simulink model "ThdRwLtStFwdBkwdTrgtPosSelc"  (R2018b)
settings: Solver=FixedStepDiscrete  StartTime=0.0  StopTime=10.0  FixedStep=0.01  RelTol=1e-3
undefined symbols (not defined in the file or in its folder): KeSMSw6sAcsEntryThdRwLtStFrwdBkwdPos_Val, KeSMSw6sAcsEntryThdRwLtStFrwdBkwdPosMax_Val, KeSMSw6sAcsEntryThdRwLtStFrwdBkwdPosMin_Val, KeSMSw6sFamilyLMdThdRwLtStFrwdBkwdPos_Val, KeSMSw6sFamilyLMdThdRwLtStFrwdBkwdPosMax_Val, KeSMSw6sFamilyLMdThdRwLtStFrwdBkwdPosMin_Val, KeSMSw6sFamilyMdThdRwLtStFrwdBkwdPos_Val, KeSMSw6sFamilyMdThdRwLtStFrwdBkwdPosMax_Val, KeSMSw6sFamilyMdThdRwLtStFrwdBkwdPosMin_Val, KeSMSw6sLugThdRwLtStFrwdBkwdPos_Val, KeSMSw6sLugThdRwLtStFrwdBkwdPosMax_Val, KeSMSw6sLugThdRwLtStFrwdBkwdPosMin_Val, KeSMSw6sVIPThdRwLtStFrwdBkwdPos_Val, KeSMSw6sVIPThdRwLtStFrwdBkwdPosMax_Val, KeSMSw6sVIPThdRwLtStFrwdBkwdPosMin_Val, KeSMSwAcsEntryThdRwLtStFrwdBkwdPos_Val, KeSMSwAcsEntryThdRwLtStFrwdBkwdPosMax_Val, KeSMSwAcsEntryThdRwLtStFrwdBkwdPosMin_Val, KeSMSwFamilyLMdThdRwLtStFrwdBkwdPos_Val, KeSMSwFamilyLMdThdRwLtStFrwdBkwdPosMax_Val, KeSMSwFamilyLMdThdRwLtStFrwdBkwdPosMin_Val, KeSMSwFamilyMdThdRwLtStFrwdBkwdPos_Val, KeSMSwFamilyMdThdRwLtStFrwdBkwdPosMax_Val, KeSMSwFamilyMdThdRwLtStFrwdBkwdPosMin_Val, KeSMSwLugThdRwLtStFrwdBkwdPos_Val, KeSMSwLugThdRwLtStFrwdBkwdPosMax_Val, KeSMSwLugThdRwLtStFrwdBkwdPosMin_Val, KeSMSwVIPThdRwLtStFrwdBkwdPos_Val, KeSMSwVIPThdRwLtStFrwdBkwdPosMax_Val, KeSMSwVIPThdRwLtStFrwdBkwdPosMin_Val
libraries: TrgtPosSelcLib x6
settings Model: Creator=sn2xws  LastModifiedBy=sn2xws
settings Model: ModifiedHistory=|
  | V2.1.0 Bug 540874 将外部标定改为固定值0
  | 2024.7.5 V3.0.0 557模式流程V1.9
settings DataIOCC: SaveFormat=StructureWithTime
settings OptimizationCC: DefaultParameterBehavior=Inlined  EnhancedBackFolding=on  PassReuseOutputArgsAs=Individual arguments  ZeroExternalMemoryAtStartup=off  ZeroInternalMemoryAtStartup=off  OptimizeBlockOrder=speed  DifferentSizesBufferReuse=on  OptimizationCustomize=off
settings DebuggingCC: ParameterTunabilityLossMsg=error
settings SFSimCC: MATLABDynamicMemAlloc=off
settings RTWCC: SystemTargetFile=autosar.tlc  GenCodeOnly=on  TemplateMakefile=ert_default_tmf  Description=AUTOSAR  GenerateReport=on  IncludeHyperlinkInReport=on  LaunchReport=on  GenerateTraceInfo=on  GenerateTraceReport=on  GenerateTraceReportSl=on  GenerateTraceReportSf=on  GenerateTraceReportEml=on  GenerateCodeMetricsReport=on
settings CodeAppCC: ForceParamTrailComments=on  IgnoreCustomStorageClasses=off  OperatorAnnotations=on  SimulinkDataObjDesc=on  SFDataObjDesc=on  InsertBlockDesc=on
settings STFCustomTargetCC: TargetLangStandard=C99 (ISO)  MultiwordLength=256  ParMdlRefBuildCompliant=on  CompOptLevelCompliant=on  IncludeMdlTerminateFcn=off  CombineOutputUpdateFcns=on  SuppressErrorStatus=on  ERTCustomFileBanners=on  SupportNonFinite=off  SupportComplex=off  SupportContinuousTime=off  SupportNonInlinedSFcns=off  RemoveResetFunc=on  MATLABClassNameForMDSCustomization=Simulink.SoftwareTarget.ERTCustomization  AutosarCompliant=on  UseToolchainInfoCompliant=on  LookupTableObjectStructAxisOrder=2,1,3,4,...  LUTObjectStructOrderEvenSpacing=Size,Table,Breakpoints  SystemTargetFile=autosar.tlc
settings ERTTargetCC: TargetLangStandard=C99 (ISO)  ConcurrentExecutionCompliant=off  IncludeMdlTerminateFcn=off  SuppressErrorStatus=on  SupportNonFinite=off  SupportComplex=off  ModelStepFunctionPrototypeControlCompliant=off  CPPClassGenCompliant=off  AutosarCompliant=on  LookupTableObjectStructAxisOrder=2,1,3,4,...  LUTObjectStructOrderEvenSpacing=Size,Table,Breakpoints  InlinedParameterPlacement=NonHierarchical  ERTCustomFileTemplate=example_file_process.tlc  ERTFilePackagingFormat=Compact

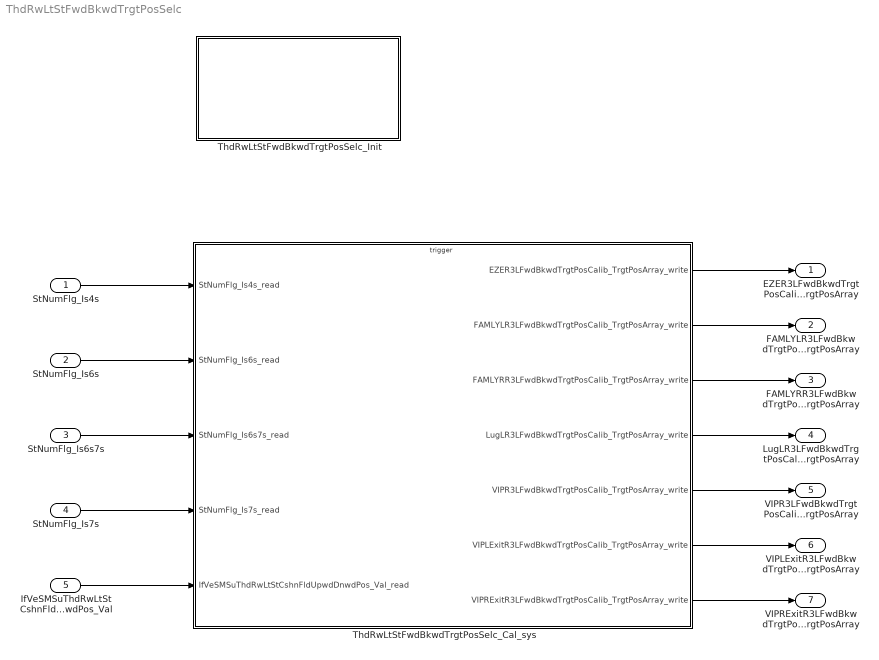
== system ThdRwLtStFwdBkwdTrgtPosSelc ==
  StNumFlg_Is4s : Inport  OutDataTypeStr=boolean  PortDimensions=1
  StNumFlg_Is6s : Inport  Port=2  OutDataTypeStr=boolean  PortDimensions=1
  StNumFlg_Is6s7s : Inport  Port=3  OutDataTypeStr=boolean  PortDimensions=1
  StNumFlg_Is7s : Inport  Port=4  OutDataTypeStr=boolean  PortDimensions=1
  IfVeSMSuThdRwLtStCshnFldUpwdDnwdPos_Val : Inport  Port=5  OutDataTypeStr=uint16  PortDimensions=1
  ThdRwLtStFwdBkwdTrgtPosSelc_Cal_sys : Subsystem
  ThdRwLtStFwdBkwdTrgtPosSelc_Init : Subsystem
  EZER3LFwdBkwdTrgtPosCalib_TrgtPosArray : Outport  Description=|  OutDataTypeStr=uint16  PortDimensions=3
      | 0:Pos
      | 1:Max
      | 2:Min
  FAMLYLR3LFwdBkwdTrgtPosCalib_TrgtPosArray : Outport  Description=|  Port=2  OutDataTypeStr=uint16  PortDimensions=3
      | 0:Pos
      | 1:Max
      | 2:Min
  FAMLYRR3LFwdBkwdTrgtPosCalib_TrgtPosArray : Outport  Description=|  Port=3  OutDataTypeStr=uint16  PortDimensions=3
      | 0:Pos
      | 1:Max
      | 2:Min
  LugLR3LFwdBkwdTrgtPosCalib_TrgtPosArray : Outport  Description=|  Port=4  OutDataTypeStr=uint16  PortDimensions=3
      | 0:Pos
      | 1:Max
      | 2:Min
  VIPR3LFwdBkwdTrgtPosCalib_TrgtPosArray : Outport  Description=|  Port=5  OutDataTypeStr=uint16  PortDimensions=3
      | 0:Pos
      | 1:Max
      | 2:Min
  VIPLExitR3LFwdBkwdTrgtPosCalib_TrgtPosArray : Outport  Description=|  Port=6  OutDataTypeStr=uint16  PortDimensions=3
      | 0:Pos
      | 1:Max
      | 2:Min
  VIPRExitR3LFwdBkwdTrgtPosCalib_TrgtPosArray : Outport  Description=|  Port=7  OutDataTypeStr=uint16  PortDimensions=3
      | 0:Pos
      | 1:Max
      | 2:Min
  wires:
  StNumFlg_Is4s/1 -> ThdRwLtStFwdBkwdTrgtPosSelc_Cal_sys/1(StNumFlg_Is4s_read)
  StNumFlg_Is6s/1 -> ThdRwLtStFwdBkwdTrgtPosSelc_Cal_sys/2(StNumFlg_Is6s_read)
  StNumFlg_Is6s7s/1 -> ThdRwLtStFwdBkwdTrgtPosSelc_Cal_sys/3(StNumFlg_Is6s7s_read)
  StNumFlg_Is7s/1 -> ThdRwLtStFwdBkwdTrgtPosSelc_Cal_sys/4(StNumFlg_Is7s_read)
  ThdRwLtStFwdBkwdTrgtPosSelc_Cal_sys/1(EZER3LFwdBkwdTrgtPosCalib_TrgtPosArray_write) -> EZER3LFwdBkwdTrgtPosCalib_TrgtPosArray/1
  ThdRwLtStFwdBkwdTrgtPosSelc_Cal_sys/2(FAMLYLR3LFwdBkwdTrgtPosCalib_TrgtPosArray_write) -> FAMLYLR3LFwdBkwdTrgtPosCalib_TrgtPosArray/1
  ThdRwLtStFwdBkwdTrgtPosSelc_Cal_sys/3(FAMLYRR3LFwdBkwdTrgtPosCalib_TrgtPosArray_write) -> FAMLYRR3LFwdBkwdTrgtPosCalib_TrgtPosArray/1
  ThdRwLtStFwdBkwdTrgtPosSelc_Cal_sys/4(LugLR3LFwdBkwdTrgtPosCalib_TrgtPosArray_write) -> LugLR3LFwdBkwdTrgtPosCalib_TrgtPosArray/1
  ThdRwLtStFwdBkwdTrgtPosSelc_Cal_sys/5(VIPR3LFwdBkwdTrgtPosCalib_TrgtPosArray_write) -> VIPR3LFwdBkwdTrgtPosCalib_TrgtPosArray/1
  ThdRwLtStFwdBkwdTrgtPosSelc_Cal_sys/6(VIPLExitR3LFwdBkwdTrgtPosCalib_TrgtPosArray_write) -> VIPLExitR3LFwdBkwdTrgtPosCalib_TrgtPosArray/1
  ThdRwLtStFwdBkwdTrgtPosSelc_Cal_sys/7(VIPRExitR3LFwdBkwdTrgtPosCalib_TrgtPosArray_write) -> VIPRExitR3LFwdBkwdTrgtPosCalib_TrgtPosArray/1
  IfVeSMSuThdRwLtStCshnFldUpwdDnwdPos_Val/1 -> ThdRwLtStFwdBkwdTrgtPosSelc_Cal_sys/5(IfVeSMSuThdRwLtStCshnFldUpwdDnwdPos_Val_read)

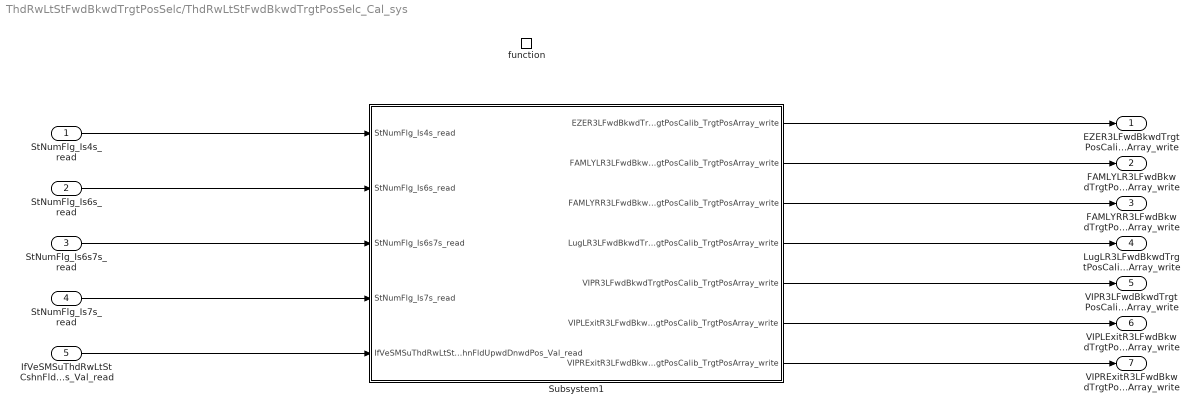
== system ThdRwLtStFwdBkwdTrgtPosSelc/ThdRwLtStFwdBkwdTrgtPosSelc_Cal_sys ==
  StNumFlg_Is4s_read : Inport
  StNumFlg_Is6s_read : Inport  Port=2
  StNumFlg_Is6s7s_read : Inport  Port=3
  StNumFlg_Is7s_read : Inport  Port=4
  IfVeSMSuThdRwLtStCshnFldUpwdDnwdPos_Val_read : Inport  Port=5
  function : TriggerPort  TriggerType=function-call  IsSimulinkFunction=on  FunctionName=ThdRwLtStFwdBkwdTrgtPosSelc_Cal  VariantControl=(inherit)
  Subsystem1 : Subsystem
  EZER3LFwdBkwdTrgtPosCalib_TrgtPosArray_write : Outport
      settings: EnsureOutportIsVirtual=on
  FAMLYLR3LFwdBkwdTrgtPosCalib_TrgtPosArray_write : Outport  Port=2
      settings: EnsureOutportIsVirtual=on
  FAMLYRR3LFwdBkwdTrgtPosCalib_TrgtPosArray_write : Outport  Port=3
      settings: EnsureOutportIsVirtual=on
  LugLR3LFwdBkwdTrgtPosCalib_TrgtPosArray_write : Outport  Port=4
      settings: EnsureOutportIsVirtual=on
  VIPR3LFwdBkwdTrgtPosCalib_TrgtPosArray_write : Outport  Port=5
      settings: EnsureOutportIsVirtual=on
  VIPLExitR3LFwdBkwdTrgtPosCalib_TrgtPosArray_write : Outport  Port=6
      settings: EnsureOutportIsVirtual=on
  VIPRExitR3LFwdBkwdTrgtPosCalib_TrgtPosArray_write : Outport  Port=7
      settings: EnsureOutportIsVirtual=on
  wires:
  Subsystem1/1(EZER3LFwdBkwdTrgtPosCalib_TrgtPosArray_write) -> EZER3LFwdBkwdTrgtPosCalib_TrgtPosArray_write/1
  Subsystem1/2(FAMLYLR3LFwdBkwdTrgtPosCalib_TrgtPosArray_write) -> FAMLYLR3LFwdBkwdTrgtPosCalib_TrgtPosArray_write/1
  Subsystem1/3(FAMLYRR3LFwdBkwdTrgtPosCalib_TrgtPosArray_write) -> FAMLYRR3LFwdBkwdTrgtPosCalib_TrgtPosArray_write/1
  Subsystem1/4(LugLR3LFwdBkwdTrgtPosCalib_TrgtPosArray_write) -> LugLR3LFwdBkwdTrgtPosCalib_TrgtPosArray_write/1
  Subsystem1/5(VIPR3LFwdBkwdTrgtPosCalib_TrgtPosArray_write) -> VIPR3LFwdBkwdTrgtPosCalib_TrgtPosArray_write/1
  StNumFlg_Is4s_read/1 -> Subsystem1/1(StNumFlg_Is4s_read)
  StNumFlg_Is6s_read/1 -> Subsystem1/2(StNumFlg_Is6s_read)
  StNumFlg_Is6s7s_read/1 -> Subsystem1/3(StNumFlg_Is6s7s_read)
  StNumFlg_Is7s_read/1 -> Subsystem1/4(StNumFlg_Is7s_read)
  Subsystem1/6(VIPLExitR3LFwdBkwdTrgtPosCalib_TrgtPosArray_write) -> VIPLExitR3LFwdBkwdTrgtPosCalib_TrgtPosArray_write/1
  Subsystem1/7(VIPRExitR3LFwdBkwdTrgtPosCalib_TrgtPosArray_write) -> VIPRExitR3LFwdBkwdTrgtPosCalib_TrgtPosArray_write/1
  IfVeSMSuThdRwLtStCshnFldUpwdDnwdPos_Val_read/1 -> Subsystem1/5(IfVeSMSuThdRwLtStCshnFldUpwdDnwdPos_Val_read)

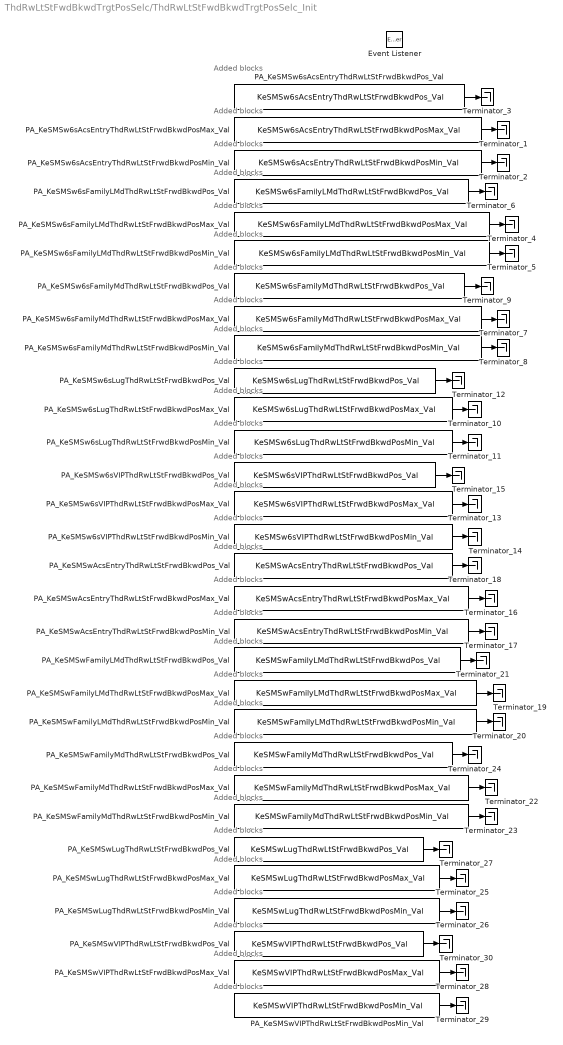
== system ThdRwLtStFwdBkwdTrgtPosSelc/ThdRwLtStFwdBkwdTrgtPosSelc_Init ==
  note: Added blocks
  note: Added blocks
  note: Added blocks
  note: Added blocks
  note: Added blocks
  note: Added blocks
  note: Added blocks
  note: Added blocks
  note: Added blocks
  note: Added blocks
  note: Added blocks
  note: Added blocks
  note: Added blocks
  note: Added blocks
  note: Added blocks
  note: Added blocks
  note: Added blocks
  note: Added blocks
  note: Added blocks
  note: Added blocks
  note: Added blocks
  note: Added blocks
  note: Added blocks
  note: Added blocks
  note: Added blocks
  note: Added blocks
  note: Added blocks
  note: Added blocks
  note: Added blocks
  note: Added blocks
  Event Listener : EventListener  EventName=reset
  PA_KeSMSw6sAcsEntryThdRwLtStFrwdBkwdPosMax_Val : Constant  Value=KeSMSw6sAcsEntryThdRwLtStFrwdBkwdPosMax_Val
  PA_KeSMSw6sAcsEntryThdRwLtStFrwdBkwdPosMin_Val : Constant  Value=KeSMSw6sAcsEntryThdRwLtStFrwdBkwdPosMin_Val
  PA_KeSMSw6sAcsEntryThdRwLtStFrwdBkwdPos_Val : Constant  Value=KeSMSw6sAcsEntryThdRwLtStFrwdBkwdPos_Val
  PA_KeSMSw6sFamilyLMdThdRwLtStFrwdBkwdPosMax_Val : Constant  Value=KeSMSw6sFamilyLMdThdRwLtStFrwdBkwdPosMax_Val
  PA_KeSMSw6sFamilyLMdThdRwLtStFrwdBkwdPosMin_Val : Constant  Value=KeSMSw6sFamilyLMdThdRwLtStFrwdBkwdPosMin_Val
  PA_KeSMSw6sFamilyLMdThdRwLtStFrwdBkwdPos_Val : Constant  Value=KeSMSw6sFamilyLMdThdRwLtStFrwdBkwdPos_Val
  PA_KeSMSw6sFamilyMdThdRwLtStFrwdBkwdPosMax_Val : Constant  Value=KeSMSw6sFamilyMdThdRwLtStFrwdBkwdPosMax_Val
  PA_KeSMSw6sFamilyMdThdRwLtStFrwdBkwdPosMin_Val : Constant  Value=KeSMSw6sFamilyMdThdRwLtStFrwdBkwdPosMin_Val
  PA_KeSMSw6sFamilyMdThdRwLtStFrwdBkwdPos_Val : Constant  Value=KeSMSw6sFamilyMdThdRwLtStFrwdBkwdPos_Val
  PA_KeSMSw6sLugThdRwLtStFrwdBkwdPosMax_Val : Constant  Value=KeSMSw6sLugThdRwLtStFrwdBkwdPosMax_Val
  PA_KeSMSw6sLugThdRwLtStFrwdBkwdPosMin_Val : Constant  Value=KeSMSw6sLugThdRwLtStFrwdBkwdPosMin_Val
  PA_KeSMSw6sLugThdRwLtStFrwdBkwdPos_Val : Constant  Value=KeSMSw6sLugThdRwLtStFrwdBkwdPos_Val
  PA_KeSMSw6sVIPThdRwLtStFrwdBkwdPosMax_Val : Constant  Value=KeSMSw6sVIPThdRwLtStFrwdBkwdPosMax_Val
  PA_KeSMSw6sVIPThdRwLtStFrwdBkwdPosMin_Val : Constant  Value=KeSMSw6sVIPThdRwLtStFrwdBkwdPosMin_Val
  PA_KeSMSw6sVIPThdRwLtStFrwdBkwdPos_Val : Constant  Value=KeSMSw6sVIPThdRwLtStFrwdBkwdPos_Val
  PA_KeSMSwAcsEntryThdRwLtStFrwdBkwdPosMax_Val : Constant  Value=KeSMSwAcsEntryThdRwLtStFrwdBkwdPosMax_Val
  PA_KeSMSwAcsEntryThdRwLtStFrwdBkwdPosMin_Val : Constant  Value=KeSMSwAcsEntryThdRwLtStFrwdBkwdPosMin_Val
  PA_KeSMSwAcsEntryThdRwLtStFrwdBkwdPos_Val : Constant  Value=KeSMSwAcsEntryThdRwLtStFrwdBkwdPos_Val
  PA_KeSMSwFamilyLMdThdRwLtStFrwdBkwdPosMax_Val : Constant  Value=KeSMSwFamilyLMdThdRwLtStFrwdBkwdPosMax_Val
  PA_KeSMSwFamilyLMdThdRwLtStFrwdBkwdPosMin_Val : Constant  Value=KeSMSwFamilyLMdThdRwLtStFrwdBkwdPosMin_Val
  PA_KeSMSwFamilyLMdThdRwLtStFrwdBkwdPos_Val : Constant  Value=KeSMSwFamilyLMdThdRwLtStFrwdBkwdPos_Val
  PA_KeSMSwFamilyMdThdRwLtStFrwdBkwdPosMax_Val : Constant  Value=KeSMSwFamilyMdThdRwLtStFrwdBkwdPosMax_Val
  PA_KeSMSwFamilyMdThdRwLtStFrwdBkwdPosMin_Val : Constant  Value=KeSMSwFamilyMdThdRwLtStFrwdBkwdPosMin_Val
  PA_KeSMSwFamilyMdThdRwLtStFrwdBkwdPos_Val : Constant  Value=KeSMSwFamilyMdThdRwLtStFrwdBkwdPos_Val
  PA_KeSMSwLugThdRwLtStFrwdBkwdPosMax_Val : Constant  Value=KeSMSwLugThdRwLtStFrwdBkwdPosMax_Val
  PA_KeSMSwLugThdRwLtStFrwdBkwdPosMin_Val : Constant  Value=KeSMSwLugThdRwLtStFrwdBkwdPosMin_Val
  PA_KeSMSwLugThdRwLtStFrwdBkwdPos_Val : Constant  Value=KeSMSwLugThdRwLtStFrwdBkwdPos_Val
  PA_KeSMSwVIPThdRwLtStFrwdBkwdPosMax_Val : Constant  Value=KeSMSwVIPThdRwLtStFrwdBkwdPosMax_Val
  PA_KeSMSwVIPThdRwLtStFrwdBkwdPosMin_Val : Constant  Value=KeSMSwVIPThdRwLtStFrwdBkwdPosMin_Val
  PA_KeSMSwVIPThdRwLtStFrwdBkwdPos_Val : Constant  Value=KeSMSwVIPThdRwLtStFrwdBkwdPos_Val
  Terminator_{1..30} (30 alike) : Terminator
  wires:
  PA_KeSMSw6sAcsEntryThdRwLtStFrwdBkwdPosMax_Val/1 -> Terminator_1/1
  PA_KeSMSw6sAcsEntryThdRwLtStFrwdBkwdPosMin_Val/1 -> Terminator_2/1
  PA_KeSMSw6sAcsEntryThdRwLtStFrwdBkwdPos_Val/1 -> Terminator_3/1
  PA_KeSMSw6sFamilyLMdThdRwLtStFrwdBkwdPosMax_Val/1 -> Terminator_4/1
  PA_KeSMSw6sFamilyLMdThdRwLtStFrwdBkwdPosMin_Val/1 -> Terminator_5/1
  PA_KeSMSw6sFamilyLMdThdRwLtStFrwdBkwdPos_Val/1 -> Terminator_6/1
  PA_KeSMSw6sFamilyMdThdRwLtStFrwdBkwdPosMax_Val/1 -> Terminator_7/1
  PA_KeSMSw6sFamilyMdThdRwLtStFrwdBkwdPosMin_Val/1 -> Terminator_8/1
  PA_KeSMSw6sFamilyMdThdRwLtStFrwdBkwdPos_Val/1 -> Terminator_9/1
  PA_KeSMSw6sLugThdRwLtStFrwdBkwdPosMax_Val/1 -> Terminator_10/1
  PA_KeSMSw6sLugThdRwLtStFrwdBkwdPosMin_Val/1 -> Terminator_11/1
  PA_KeSMSw6sLugThdRwLtStFrwdBkwdPos_Val/1 -> Terminator_12/1
  PA_KeSMSw6sVIPThdRwLtStFrwdBkwdPosMax_Val/1 -> Terminator_13/1
  PA_KeSMSw6sVIPThdRwLtStFrwdBkwdPosMin_Val/1 -> Terminator_14/1
  PA_KeSMSw6sVIPThdRwLtStFrwdBkwdPos_Val/1 -> Terminator_15/1
  PA_KeSMSwAcsEntryThdRwLtStFrwdBkwdPosMax_Val/1 -> Terminator_16/1
  PA_KeSMSwAcsEntryThdRwLtStFrwdBkwdPosMin_Val/1 -> Terminator_17/1
  PA_KeSMSwAcsEntryThdRwLtStFrwdBkwdPos_Val/1 -> Terminator_18/1
  PA_KeSMSwFamilyLMdThdRwLtStFrwdBkwdPosMax_Val/1 -> Terminator_19/1
  PA_KeSMSwFamilyLMdThdRwLtStFrwdBkwdPosMin_Val/1 -> Terminator_20/1
  PA_KeSMSwFamilyLMdThdRwLtStFrwdBkwdPos_Val/1 -> Terminator_21/1
  PA_KeSMSwFamilyMdThdRwLtStFrwdBkwdPosMax_Val/1 -> Terminator_22/1
  PA_KeSMSwFamilyMdThdRwLtStFrwdBkwdPosMin_Val/1 -> Terminator_23/1
  PA_KeSMSwFamilyMdThdRwLtStFrwdBkwdPos_Val/1 -> Terminator_24/1
  PA_KeSMSwLugThdRwLtStFrwdBkwdPosMax_Val/1 -> Terminator_25/1
  PA_KeSMSwLugThdRwLtStFrwdBkwdPosMin_Val/1 -> Terminator_26/1
  PA_KeSMSwLugThdRwLtStFrwdBkwdPos_Val/1 -> Terminator_27/1
  PA_KeSMSwVIPThdRwLtStFrwdBkwdPosMax_Val/1 -> Terminator_28/1
  PA_KeSMSwVIPThdRwLtStFrwdBkwdPosMin_Val/1 -> Terminator_29/1
  PA_KeSMSwVIPThdRwLtStFrwdBkwdPos_Val/1 -> Terminator_30/1

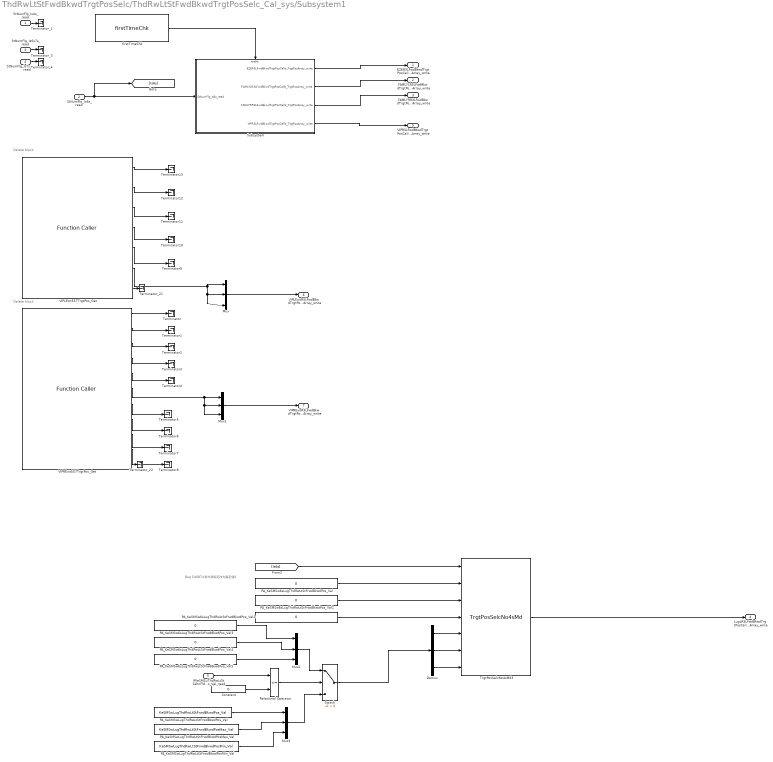
== system ThdRwLtStFwdBkwdTrgtPosSelc/ThdRwLtStFwdBkwdTrgtPosSelc_Cal_sys/Subsystem1 ==
  note: Delete block
  note: Delete block
  note: Bug 540874 将外部标定改为固定值0
  StNumFlg_Is4s_read : Inport
  StNumFlg_Is6s_read : Inport  Port=2
  StNumFlg_Is6s7s_read : Inport  Port=3
  StNumFlg_Is7s_read : Inport  Port=4
  IfVeSMSuThdRwLtStCshnFldUpwdDnwdPos_Val_read : Inport  Port=5
  Constant : Constant  Value=0  OutDataTypeStr=uint16
  Demux : Demux  Outputs=3
  Mux{,1..3} (4 alike) : Mux  Inputs=3
  PA_KeSMSw6sLugThdRwLtStFrwdBkwdPos_Val{,1..5} (6 alike) : Constant  Value=0  OutDataTypeStr=uint16
  PA_KeSMSwLugThdRwLtStFrwdBkwdPosMax_Val : Constant  Value=KeSMSwLugThdRwLtStFrwdBkwdPosMax_Val
  PA_KeSMSwLugThdRwLtStFrwdBkwdPosMin_Val : Constant  Value=KeSMSwLugThdRwLtStFrwdBkwdPosMin_Val
  PA_KeSMSwLugThdRwLtStFrwdBkwdPos_Val : Constant  Value=KeSMSwLugThdRwLtStFrwdBkwdPos_Val
  Relational Operator : RelationalOperator  Operator=<=  OutDataTypeStr=boolean  RndMeth=Simplest
  Subsystem : Subsystem
  Switch : Switch  Criteria=u2 > Threshold
  Terminator{,1..13} (14 alike) : Terminator
  Terminator_{1,3..4,21..22} (5 alike) : Terminator
  TrgtPosSelcNo4sMd3 : TrgtPosSelcLib/TrgtPosSelcNo4sMd  SystemSampleTime=-1
  VIPLExit557TrgtPos_Get : FunctionCaller  FunctionPrototype=[SecRwLtStBkReclnTrgtPos,SecRwLtStZeroTrgtPos,SecRwLtStLgrstUpwdDnwdTrgtPos,SecRwLtStLgrstInwdOtwdTrgtPos,ThdRwLtStBkReclnTrgtPos,ThdRwLtStFwdBkwdTrgtPos,SecRwLtStFwdBkwdTrgtPos] = VIPLExit557TrgtPos_Get()  OutputArgumentSpecifications=uint16(1), uint16(1), uint16(1), uint16(1), uint16(1), uint16(1), uint16(1)
  VIPRExit557TrgtPos_Get : FunctionCaller  FunctionPrototype=[SecRwRtStBkReclnTrgtPos,SecRwRtStZeroTrgtPos,SecRwRtStLgrstUpwdDnwdTrgtPos,SecRwRtStLgrstInwdOtwdTrgtPos,ThdRwLtStBkReclnTrgtPos,ThdRwLtStFwdBkwdTrgtPos,ThdRwRtStBkReclnTrgtPos,ThdRwRtStFwdBkwdTrgtPos,PassStBkReclnTrgtPos,PassStFwdBkwdTrgtPos,SecRwRtStFwdBkwdTrgtPos] = VIPRExit557TrgtPos_Get()  OutputArgumentSpecifications=uint16(1), uint16(1), uint16(1), uint16(1), uint16(1), uint16(1), uint16(1), uint16(1), uint16(1), uint16(1), uint16(1)
  firstTimeChk : TrgtPosSelcLib/firstTimeChk  SystemSampleTime=-1
  EZER3LFwdBkwdTrgtPosCalib_TrgtPosArray_write : Outport
      settings: EnsureOutportIsVirtual=on
  FAMLYLR3LFwdBkwdTrgtPosCalib_TrgtPosArray_write : Outport  Port=2
      settings: EnsureOutportIsVirtual=on
  FAMLYRR3LFwdBkwdTrgtPosCalib_TrgtPosArray_write : Outport  Port=3
      settings: EnsureOutportIsVirtual=on
  LugLR3LFwdBkwdTrgtPosCalib_TrgtPosArray_write : Outport  Port=4
      settings: EnsureOutportIsVirtual=on
  VIPR3LFwdBkwdTrgtPosCalib_TrgtPosArray_write : Outport  Port=5
      settings: EnsureOutportIsVirtual=on
  VIPLExitR3LFwdBkwdTrgtPosCalib_TrgtPosArray_write : Outport  Port=6
      settings: EnsureOutportIsVirtual=on
  VIPRExitR3LFwdBkwdTrgtPosCalib_TrgtPosArray_write : Outport  Port=7
      settings: EnsureOutportIsVirtual=on
  wires:
  Subsystem/4(VIPR3LFwdBkwdTrgtPosCalib_TrgtPosArray_write) -> VIPR3LFwdBkwdTrgtPosCalib_TrgtPosArray_write/1
  StNumFlg_Is7s_read/1 -> Terminator_4/1
  TrgtPosSelcNo4sMd3/1 -> LugLR3LFwdBkwdTrgtPosCalib_TrgtPosArray_write/1
  StNumFlg_Is4s_read/1 -> Terminator_1/1
  Subsystem/2(FAMLYLR3LFwdBkwdTrgtPosCalib_TrgtPosArray_write) -> FAMLYLR3LFwdBkwdTrgtPosCalib_TrgtPosArray_write/1
  Subsystem/3(FAMLYRR3LFwdBkwdTrgtPosCalib_TrgtPosArray_write) -> FAMLYRR3LFwdBkwdTrgtPosCalib_TrgtPosArray_write/1
  Subsystem/1(EZER3LFwdBkwdTrgtPosCalib_TrgtPosArray_write) -> EZER3LFwdBkwdTrgtPosCalib_TrgtPosArray_write/1
  firstTimeChk/1 -> Subsystem/Enable
  StNumFlg_Is6s_read/1 -> [Is6s], Subsystem/1(StNumFlg_Is6s_read)
  StNumFlg_Is6s7s_read/1 -> Terminator_3/1
  Mux/1 -> VIPLExitR3LFwdBkwdTrgtPosCalib_TrgtPosArray_write/1
  VIPLExit557TrgtPos_Get/6 -> Mux/3, Mux/2, Mux/1
  VIPRExit557TrgtPos_Get/6 -> Mux1/1, Mux1/2, Mux1/3
  Mux1/1 -> VIPRExitR3LFwdBkwdTrgtPosCalib_TrgtPosArray_write/1
  VIPRExit557TrgtPos_Get/1 -> Terminator/1
  VIPRExit557TrgtPos_Get/2 -> Terminator1/1
  VIPRExit557TrgtPos_Get/3 -> Terminator2/1
  VIPRExit557TrgtPos_Get/4 -> Terminator3/1
  VIPRExit557TrgtPos_Get/5 -> Terminator4/1
  VIPRExit557TrgtPos_Get/7 -> Terminator5/1
  VIPRExit557TrgtPos_Get/8 -> Terminator6/1
  VIPRExit557TrgtPos_Get/9 -> Terminator7/1
  VIPRExit557TrgtPos_Get/10 -> Terminator8/1
  VIPLExit557TrgtPos_Get/5 -> Terminator9/1
  VIPLExit557TrgtPos_Get/4 -> Terminator10/1
  VIPLExit557TrgtPos_Get/3 -> Terminator11/1
  VIPLExit557TrgtPos_Get/2 -> Terminator12/1
  VIPLExit557TrgtPos_Get/1 -> Terminator13/1
  PA_KeSMSw6sLugThdRwLtStFrwdBkwdPos_Val2/1 -> TrgtPosSelcNo4sMd3/4
  PA_KeSMSw6sLugThdRwLtStFrwdBkwdPos_Val1/1 -> TrgtPosSelcNo4sMd3/3
  PA_KeSMSw6sLugThdRwLtStFrwdBkwdPos_Val/1 -> TrgtPosSelcNo4sMd3/2
  [Is6s] -> TrgtPosSelcNo4sMd3/1
  VIPLExit557TrgtPos_Get/7 -> Terminator_21/1
  VIPRExit557TrgtPos_Get/11 -> Terminator_22/1
  IfVeSMSuThdRwLtStCshnFldUpwdDnwdPos_Val_read/1 -> Relational Operator/1
  Constant/1 -> Relational Operator/2
  Relational Operator/1 -> Switch/2
  Mux2/1 -> Switch/1
  PA_KeSMSw6sLugThdRwLtStFrwdBkwdPos_Val3/1 -> Mux2/1
  PA_KeSMSw6sLugThdRwLtStFrwdBkwdPos_Val4/1 -> Mux2/2
  PA_KeSMSw6sLugThdRwLtStFrwdBkwdPos_Val5/1 -> Mux2/3
  PA_KeSMSwLugThdRwLtStFrwdBkwdPos_Val/1 -> Mux3/1
  PA_KeSMSwLugThdRwLtStFrwdBkwdPosMax_Val/1 -> Mux3/2
  PA_KeSMSwLugThdRwLtStFrwdBkwdPosMin_Val/1 -> Mux3/3
  Mux3/1 -> Switch/3
  Switch/1 -> Demux/1
  Demux/1 -> TrgtPosSelcNo4sMd3/5
  Demux/2 -> TrgtPosSelcNo4sMd3/6
  Demux/3 -> TrgtPosSelcNo4sMd3/7

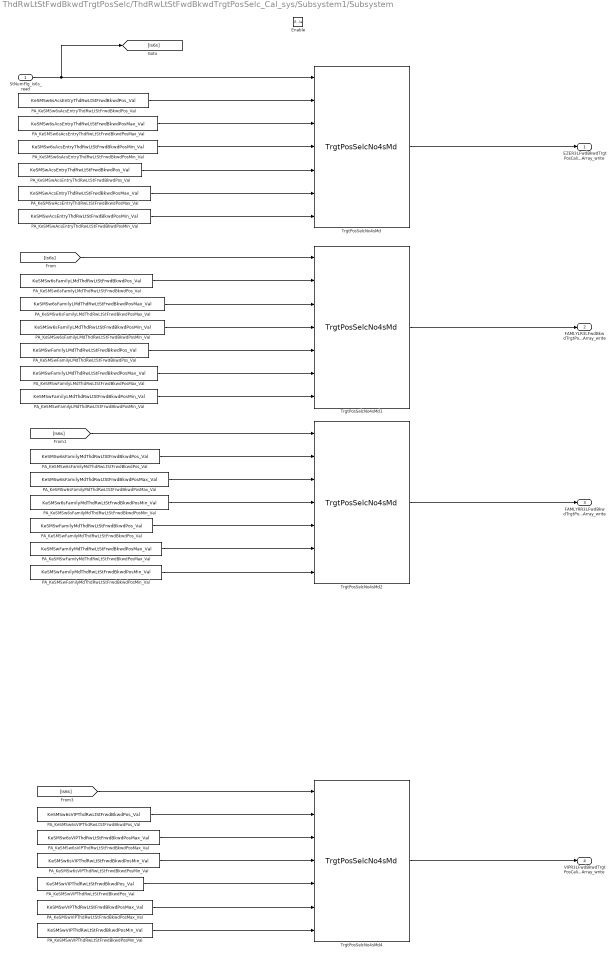
== system ThdRwLtStFwdBkwdTrgtPosSelc/ThdRwLtStFwdBkwdTrgtPosSelc_Cal_sys/Subsystem1/Subsystem ==
  StNumFlg_Is6s_read : Inport
  Enable : EnablePort
  PA_KeSMSw6sAcsEntryThdRwLtStFrwdBkwdPosMax_Val : Constant  Value=KeSMSw6sAcsEntryThdRwLtStFrwdBkwdPosMax_Val
  PA_KeSMSw6sAcsEntryThdRwLtStFrwdBkwdPosMin_Val : Constant  Value=KeSMSw6sAcsEntryThdRwLtStFrwdBkwdPosMin_Val
  PA_KeSMSw6sAcsEntryThdRwLtStFrwdBkwdPos_Val : Constant  Value=KeSMSw6sAcsEntryThdRwLtStFrwdBkwdPos_Val
  PA_KeSMSw6sFamilyLMdThdRwLtStFrwdBkwdPosMax_Val : Constant  Value=KeSMSw6sFamilyLMdThdRwLtStFrwdBkwdPosMax_Val
  PA_KeSMSw6sFamilyLMdThdRwLtStFrwdBkwdPosMin_Val : Constant  Value=KeSMSw6sFamilyLMdThdRwLtStFrwdBkwdPosMin_Val
  PA_KeSMSw6sFamilyLMdThdRwLtStFrwdBkwdPos_Val : Constant  Value=KeSMSw6sFamilyLMdThdRwLtStFrwdBkwdPos_Val
  PA_KeSMSw6sFamilyMdThdRwLtStFrwdBkwdPosMax_Val : Constant  Value=KeSMSw6sFamilyMdThdRwLtStFrwdBkwdPosMax_Val
  PA_KeSMSw6sFamilyMdThdRwLtStFrwdBkwdPosMin_Val : Constant  Value=KeSMSw6sFamilyMdThdRwLtStFrwdBkwdPosMin_Val
  PA_KeSMSw6sFamilyMdThdRwLtStFrwdBkwdPos_Val : Constant  Value=KeSMSw6sFamilyMdThdRwLtStFrwdBkwdPos_Val
  PA_KeSMSw6sVIPThdRwLtStFrwdBkwdPosMax_Val : Constant  Value=KeSMSw6sVIPThdRwLtStFrwdBkwdPosMax_Val
  PA_KeSMSw6sVIPThdRwLtStFrwdBkwdPosMin_Val : Constant  Value=KeSMSw6sVIPThdRwLtStFrwdBkwdPosMin_Val
  PA_KeSMSw6sVIPThdRwLtStFrwdBkwdPos_Val : Constant  Value=KeSMSw6sVIPThdRwLtStFrwdBkwdPos_Val
  PA_KeSMSwAcsEntryThdRwLtStFrwdBkwdPosMax_Val : Constant  Value=KeSMSwAcsEntryThdRwLtStFrwdBkwdPosMax_Val
  PA_KeSMSwAcsEntryThdRwLtStFrwdBkwdPosMin_Val : Constant  Value=KeSMSwAcsEntryThdRwLtStFrwdBkwdPosMin_Val
  PA_KeSMSwAcsEntryThdRwLtStFrwdBkwdPos_Val : Constant  Value=KeSMSwAcsEntryThdRwLtStFrwdBkwdPos_Val
  PA_KeSMSwFamilyLMdThdRwLtStFrwdBkwdPosMax_Val : Constant  Value=KeSMSwFamilyLMdThdRwLtStFrwdBkwdPosMax_Val
  PA_KeSMSwFamilyLMdThdRwLtStFrwdBkwdPosMin_Val : Constant  Value=KeSMSwFamilyLMdThdRwLtStFrwdBkwdPosMin_Val
  PA_KeSMSwFamilyLMdThdRwLtStFrwdBkwdPos_Val : Constant  Value=KeSMSwFamilyLMdThdRwLtStFrwdBkwdPos_Val
  PA_KeSMSwFamilyMdThdRwLtStFrwdBkwdPosMax_Val : Constant  Value=KeSMSwFamilyMdThdRwLtStFrwdBkwdPosMax_Val
  PA_KeSMSwFamilyMdThdRwLtStFrwdBkwdPosMin_Val : Constant  Value=KeSMSwFamilyMdThdRwLtStFrwdBkwdPosMin_Val
  PA_KeSMSwFamilyMdThdRwLtStFrwdBkwdPos_Val : Constant  Value=KeSMSwFamilyMdThdRwLtStFrwdBkwdPos_Val
  PA_KeSMSwVIPThdRwLtStFrwdBkwdPosMax_Val : Constant  Value=KeSMSwVIPThdRwLtStFrwdBkwdPosMax_Val
  PA_KeSMSwVIPThdRwLtStFrwdBkwdPosMin_Val : Constant  Value=KeSMSwVIPThdRwLtStFrwdBkwdPosMin_Val
  PA_KeSMSwVIPThdRwLtStFrwdBkwdPos_Val : Constant  Value=KeSMSwVIPThdRwLtStFrwdBkwdPos_Val
  TrgtPosSelcNo4sMd{,1..2,4} (4 alike) : TrgtPosSelcLib/TrgtPosSelcNo4sMd  SystemSampleTime=-1
  EZER3LFwdBkwdTrgtPosCalib_TrgtPosArray_write : Outport
      settings: EnsureOutportIsVirtual=on
  FAMLYLR3LFwdBkwdTrgtPosCalib_TrgtPosArray_write : Outport  Port=2
      settings: EnsureOutportIsVirtual=on
  FAMLYRR3LFwdBkwdTrgtPosCalib_TrgtPosArray_write : Outport  Port=3
      settings: EnsureOutportIsVirtual=on
  VIPR3LFwdBkwdTrgtPosCalib_TrgtPosArray_write : Outport  Port=4
      settings: EnsureOutportIsVirtual=on
  wires:
  StNumFlg_Is6s_read/1 -> [Is6s], TrgtPosSelcNo4sMd/1
  TrgtPosSelcNo4sMd/1 -> EZER3LFwdBkwdTrgtPosCalib_TrgtPosArray_write/1
  TrgtPosSelcNo4sMd1/1 -> FAMLYLR3LFwdBkwdTrgtPosCalib_TrgtPosArray_write/1
  TrgtPosSelcNo4sMd2/1 -> FAMLYRR3LFwdBkwdTrgtPosCalib_TrgtPosArray_write/1
  TrgtPosSelcNo4sMd4/1 -> VIPR3LFwdBkwdTrgtPosCalib_TrgtPosArray_write/1
  PA_KeSMSw6sAcsEntryThdRwLtStFrwdBkwdPosMax_Val/1 -> TrgtPosSelcNo4sMd/3
  PA_KeSMSw6sAcsEntryThdRwLtStFrwdBkwdPosMin_Val/1 -> TrgtPosSelcNo4sMd/4
  PA_KeSMSw6sAcsEntryThdRwLtStFrwdBkwdPos_Val/1 -> TrgtPosSelcNo4sMd/2
  [Is6s] -> TrgtPosSelcNo4sMd1/1
  PA_KeSMSw6sFamilyLMdThdRwLtStFrwdBkwdPosMax_Val/1 -> TrgtPosSelcNo4sMd1/3
  PA_KeSMSw6sFamilyLMdThdRwLtStFrwdBkwdPosMin_Val/1 -> TrgtPosSelcNo4sMd1/4
  PA_KeSMSw6sFamilyLMdThdRwLtStFrwdBkwdPos_Val/1 -> TrgtPosSelcNo4sMd1/2
  [Is6s] -> TrgtPosSelcNo4sMd2/1
  [Is6s] -> TrgtPosSelcNo4sMd4/1
  PA_KeSMSw6sFamilyMdThdRwLtStFrwdBkwdPosMax_Val/1 -> TrgtPosSelcNo4sMd2/3
  PA_KeSMSw6sFamilyMdThdRwLtStFrwdBkwdPosMin_Val/1 -> TrgtPosSelcNo4sMd2/4
  PA_KeSMSw6sFamilyMdThdRwLtStFrwdBkwdPos_Val/1 -> TrgtPosSelcNo4sMd2/2
  PA_KeSMSw6sVIPThdRwLtStFrwdBkwdPosMax_Val/1 -> TrgtPosSelcNo4sMd4/3
  PA_KeSMSw6sVIPThdRwLtStFrwdBkwdPos_Val/1 -> TrgtPosSelcNo4sMd4/2
  PA_KeSMSw6sVIPThdRwLtStFrwdBkwdPosMin_Val/1 -> TrgtPosSelcNo4sMd4/4
  PA_KeSMSwAcsEntryThdRwLtStFrwdBkwdPosMax_Val/1 -> TrgtPosSelcNo4sMd/6
  PA_KeSMSwAcsEntryThdRwLtStFrwdBkwdPos_Val/1 -> TrgtPosSelcNo4sMd/5
  PA_KeSMSwAcsEntryThdRwLtStFrwdBkwdPosMin_Val/1 -> TrgtPosSelcNo4sMd/7
  PA_KeSMSwFamilyLMdThdRwLtStFrwdBkwdPosMax_Val/1 -> TrgtPosSelcNo4sMd1/6
  PA_KeSMSwFamilyLMdThdRwLtStFrwdBkwdPosMin_Val/1 -> TrgtPosSelcNo4sMd1/7
  PA_KeSMSwFamilyLMdThdRwLtStFrwdBkwdPos_Val/1 -> TrgtPosSelcNo4sMd1/5
  PA_KeSMSwFamilyMdThdRwLtStFrwdBkwdPosMax_Val/1 -> TrgtPosSelcNo4sMd2/6
  PA_KeSMSwFamilyMdThdRwLtStFrwdBkwdPosMin_Val/1 -> TrgtPosSelcNo4sMd2/7
  PA_KeSMSwFamilyMdThdRwLtStFrwdBkwdPos_Val/1 -> TrgtPosSelcNo4sMd2/5
  PA_KeSMSwVIPThdRwLtStFrwdBkwdPosMax_Val/1 -> TrgtPosSelcNo4sMd4/6
  PA_KeSMSwVIPThdRwLtStFrwdBkwdPos_Val/1 -> TrgtPosSelcNo4sMd4/5
  PA_KeSMSwVIPThdRwLtStFrwdBkwdPosMin_Val/1 -> TrgtPosSelcNo4sMd4/7
